simulink model "transfer_function_calculation"  (R2016a)
settings: Solver=VariableStepAuto  StartTime=0.0  StopTime=5  RelTol=1e-3
values from neighbouring files (symbols this model uses):
  a = .7    (= 0.7)    [PM_1_5MW_syn_27.m]
  Flux = 5.8264    [PM_1_5MW_syn_27.m]
  Id_set = 500    [PM_1_5MW_syn_27.m]
  Iq_set = -2200    [PM_1_5MW_syn_27.m]
  L = .0001    (= 0.0001)    [PM_1_5MW_syn_27.m]
  Ld = 0.001575    [PM_1_5MW_syn_27.m]
  Lq = 0.001575    [PM_1_5MW_syn_27.m]
  mn = 60000    [PM_1_5MW_syn_27.m]
  p = 26    [PM_1_5MW_syn_27.m]
  Rs = 0.000821    [PM_1_5MW_syn_27.m]
  Sollkurve_M_Optimum = [0 57121 101549 158670 228485 310994 406196 514092 634681 767965 810425 823386 ... (13 elements, 13x1)]    [Lookup_M_n.mat]
  Sollkurve_nGen_Optimum = [0 5 7 9 11 12 14 16 18 20 20.07 20.2 ... (13 elements, 13x1)]    [Lookup_M_n.mat]
  Speed_set = w_m    (= 2.10172548525)    [PM_1_5MW_syn_27.m]
  Ts_Power = 5.000000000000000e-06    (= 5e-06)    [PM_1_5MW_syn_27.m]
  Vdc = 1200    [PM_1_5MW_syn_27.m]
  Vh = Vm/6*0    (= 0)    [PM_1_5MW_syn_27.m]
undefined symbols (not defined in the file or in its folder): C2, Esw_Erec, Esw_Off, Esw_On, Page_Temp_C
undefined symbols (not defined in the file): Ts_Control, z
libraries: fl_lib x84, powerlib_meascontrol x58, simulink x56, nesl_utility x36, powerlib x33, simulink_extras x11
(part 3 of 6)

== system transfer_function_calculation/Generator/Generator /power calculation ==
  vdq : Inport
  idq : Inport  Port=2
  Complex to Magnitude-Angle : ComplexToMagnitudeAngle
  Complex to Real-Imag : ComplexToRealImag
  Demux : Demux  Outputs=2
  Demux1 : Demux  Outputs=2
  Gain : Gain  Gain=180/pi
  Gain1 : Gain  Gain=-1
  Gain4 : Gain  Gain=3/2
  Product2 : Product  RndMeth=Zero
  Real-Imag to Complex : RealImagToComplex
  Real-Imag to Complex1 : RealImagToComplex
  Trigonometric Function : Trigonometry  Operator=cos
  apparent power : Outport
  active power : Outport  Port=2
  reactive power : Outport  Port=3
  phi : Outport  Port=4
  cos phi : Outport  Port=5
  wires:
  Demux/1 -> Real-Imag to Complex/1
  Demux/2 -> Real-Imag to Complex/2
  Demux1/1 -> Real-Imag to Complex1/1
  Real-Imag to Complex/1 -> Product2/1
  Real-Imag to Complex1/1 -> Product2/2
  Product2/1 -> Gain4/1
  vdq/1 -> Demux/1
  idq/1 -> Demux1/1
  Complex to Magnitude-Angle/1 -> apparent power/1
  Complex to Magnitude-Angle/2 -> Trigonometric Function/1, Gain/1
  Gain/1 -> phi/1
  Demux1/2 -> Gain1/1
  Gain1/1 -> Real-Imag to Complex1/2
  Trigonometric Function/1 -> cos phi/1
  Complex to Real-Imag/1 -> active power/1
  Complex to Real-Imag/2 -> reactive power/1
  Gain4/1 -> Complex to Real-Imag/1, Complex to Magnitude-Angle/1

== system transfer_function_calculation/Generator/Generator Controller /Id controller ==
  Id_set : Inport
  Id_meas : Inport  Port=2
  Step : Step  Before=1  SampleTime=0
  Sum2 : Sum  Inputs=|-+
  Transfer Fcn (with initial states)1 : simulink_extras/Additional Linear/Transfer Fcn (with initial states)  N=[1 2888 714941]*7.50  D=[1 5626 5375320]  X0=0
  id : Scope  NumInputPorts=2
  id1 : Scope
  Vd_ref : Outport
  wires:
  Id_set/1 -> id/2, id1/1, Sum2/2
  Sum2/1 -> Transfer Fcn (with initial states)1/1
  Id_meas/1 -> id/1, Sum2/1
  Transfer Fcn (with initial states)1/1 -> Vd_ref/1

== system transfer_function_calculation/Generator/Generator Controller /Inverse Clarke Transformation ==
  ab : Inport
  Demux : Demux  Outputs=2
  Gain1 : Gain  Gain=1/2
  Gain2 : Gain  Gain=sqrt(3)
  Gain4 : Gain  Gain=1/2
  Mux : Mux  Inputs=3
  Sum : Sum  Inputs=|-+
  Sum1 : Sum  Inputs=|--
  abc : Outport
  wires:
  Mux/1 -> abc/1
  ab/1 -> Demux/1
  Sum1/1 -> Gain1/1
  Sum/1 -> Gain4/1
  Gain2/1 -> Sum1/2, Sum/2
  Demux/1 -> Sum1/1, Sum/1, Mux/1
  Demux/2 -> Gain2/1
  Gain4/1 -> Mux/2
  Gain1/1 -> Mux/3

== system transfer_function_calculation/Generator/Generator Controller /Inverse Park Transformation ==
  dq : Inport
  angle : Inport  Port=2
  Demux : Demux  Outputs=2
  Mux : Mux  Inputs=2
  Product{,1..3} (4 alike) : Product  RndMeth=Zero
  Sum : Sum  Inputs=|+-
  Sum1 : Sum  Inputs=|++
  cosine : Trigonometry  Operator=cos
  sine : Trigonometry
  ab : Outport
  wires:
  Sum1/1 -> Mux/2
  Sum/1 -> Mux/1
  Product2/1 -> Sum/2
  Product1/1 -> Sum/1
  Product3/1 -> Sum1/2
  Product/1 -> Sum1/1
  angle/1 -> cosine/1, sine/1
  cosine/1 -> Product3/2, Product1/2
  sine/1 -> Product2/2, Product/2
  Demux/2 -> Product3/1, Product2/1
  Demux/1 -> Product1/1, Product/1
  Mux/1 -> ab/1
  dq/1 -> Demux/1

== system transfer_function_calculation/Generator/Generator Controller /Iq controller ==
  Iq_meas : Inport
  Iq_set : Inport  Port=2
  Sum1 : Sum  Inputs=|-+
  Transfer Fcn (with initial states)1 : simulink_extras/Additional Linear/Transfer Fcn (with initial states)  N=[1 2888 714941]*7.50  D=[1 5626 5375320]  X0=0
  iq : Scope  NumInputPorts=2
  iq1 : Scope
  Vq_ref : Outport
  wires:
  Iq_set/1 -> iq/1, Sum1/2
  Sum1/1 -> Transfer Fcn (with initial states)1/1
  Iq_meas/1 -> iq1/1, iq/2, Sum1/1
  Transfer Fcn (with initial states)1/1 -> Vq_ref/1

== system transfer_function_calculation/Generator/Generator Controller /Parktransformation ==
  i_abc : Inport
  theta : Inport  Port=2
  3phase to ab : Subsystem
  Cartesian to Polar : simulink_extras/Transformations/Cartesian to Polar
  Demux : Demux  Outputs=2
  Display : Display
  Display1 : Display
  Scope : Scope  NumInputPorts=3
  Scope1 : Scope  NumInputPorts=3
  Scope2 : Scope  NumInputPorts=3
  alpha-beta to dq : Subsystem
  i_dq : Outport
  wires:
  3phase to ab/1(Out1) -> Scope/2, Demux/1, alpha-beta to dq/2("alpha-beta ")
  alpha-beta to dq/1(Out1) -> Scope/1, i_dq/1
  i_abc/1 -> Scope1/1, 3phase to ab/1(In1)
  theta/1 -> Scope/3, alpha-beta to dq/1(theta)
  Demux/1 -> Cartesian to Polar/1
  Demux/2 -> Cartesian to Polar/2
  Cartesian to Polar/1 -> Scope2/1, Display/1
  Cartesian to Polar/2 -> Scope2/2, Display1/1

== system transfer_function_calculation/Generator/Generator Controller /Speed Controller ==
  meas : Inport
  set : Inport  Port=2
  PID Controller1 : simulink/Continuous/PID Controller  Controller=PI  TimeDomain=Continuous-time  SampleTime=-1  IntegratorMethod=Forward Euler  FilterMethod=Forward Euler  Form=Parallel  UseFilter=on  ControllerParametersSource=internal  P=5437  I=1000000  D=0  N=100  InitialConditionSource=internal  InitialConditionForIntegrator=0  InitialConditionForFilter=0  ExternalReset=none  LimitOutput=off  UpperSaturationLimit=inf  LowerSaturationLimit=-inf  LinearizeAsGain=on  AntiWindupMode=none  Kb=1  TrackingMode=off  Kt=1  PParamMin=[]  PParamMax=[]  IParamMin=[]  IParamMax=[]  DParamMin=[]  DParamMax=[]  NParamMin=[]  NParamMax=[]  KbParamMin=[]  KbParamMax=[]  KtParamMin=[]  KtParamMax=[]  POutMin=[]  POutMax=[]  IOutMin=[]  IOutMax=[]  DOutMin=[]  DOutMax=[]  NOutMin=[]  NOutMax=[]  KbOutMin=[]  KbOutMax=[]  KtOutMin=[]  KtOutMax=[]  IntegratorOutMin=[]  IntegratorOutMax=[]  FilterOutMin=[]  FilterOutMax=[]  SumOutMin=[]  SumOutMax=[]  SumI1OutMin=[]  SumI1OutMax=[]  SumI2OutMin=[]  SumI2OutMax=[]  SumI3OutMin=[]  SumI3OutMax=[]  SumDOutMin=[]  SumDOutMax=[]  SaturationOutMin=[]  SaturationOutMax=[]  IntegratorContinuousStateAttributes=''  IntegratorStateMustResolveToSignalObject=off  IntegratorRTWStateStorageClass=Auto  FilterContinuousStateAttributes=''  FilterStateMustResolveToSignalObject=off  FilterRTWStateStorageClass=Auto  DifferentiatorICPrevScaledInput=0  DifferentiatorOutMin=[]  DifferentiatorOutMax=[]
  Sum1 : Sum  Inputs=|-+
  Transfer Fcn (with initial states)1 : simulink_extras/Additional Linear/Transfer Fcn (with initial states)  Commented=on  N=[18.688 3793]  D=[1 3808]  X0=0
  "speed " : Scope  NumInputPorts=2
  speed 1 : Scope
  Act : Outport
  wires:
  set/1 -> "speed "/1, Sum1/2
  meas/1 -> "speed "/2, speed 1/1, Sum1/1
  Sum1/1 -> PID Controller1/1
  PID Controller1/1 -> Act/1

== system transfer_function_calculation/Generator/Modulation index2/Clarke transformation ==
  In1 : Inport
  Demux : Demux  Outputs=3
  Gain3 : Gain  Gain=1/sqrt(3)
  Mux : Mux  Inputs=2
  Scope : Scope
  Sum1 : Sum  Inputs=|+-
  Out1 : Outport
  wires:
  Gain3/1 -> Mux/2
  Demux/1 -> Mux/1
  In1/1 -> Demux/1
  Sum1/1 -> Gain3/1
  Demux/3 -> Sum1/2
  Demux/2 -> Sum1/1
  Mux/1 -> Out1/1, Scope/1

== system transfer_function_calculation/Generator/3 Level Converter2/Loss Calculation/Leg A1 ==
  G : Inport  PortDimensions=2
  G1 : Inport  Port=2  PortDimensions=2
  Ambient Temperature (C) : Constant  Value=40
  Heat Sink (Simscape thermal model) : Subsystem  mask(Simscape Thermal model (2-cell Cauer network)){Rth=[ 0.02  0.072 ], Cth=[ 5  10 ]/10, Tinit=123}
      mask prompts: Rth "Thermal resistances  [case-to-sink  sink-to-ambient ] (K/W):"; Cth "Thermal capacitances  [case  sink ] (J/K):"; Tinit "Initial temperature (degrees Celsisus)"
  Scope : Scope
  Scope1 : Scope
  Subsystem : Subsystem
  Tsink : Scope
  m : Outport
  wires:
  G/1 -> Subsystem/1(In1), Scope/1
  G1/1 -> Scope1/1, Subsystem/2(In2)
  Ambient Temperature (C)/1 -> Heat Sink (Simscape thermal model)/1(Ta)
  Heat Sink (Simscape thermal model)/1(Tsink) -> Tsink/1
  Subsystem/1(Out1) -> m/1
  connections:
  Heat Sink (Simscape thermal model)/RConn1 -- Subsystem/LConn1

== system transfer_function_calculation/Generator/3 Level Converter2/Loss Calculation/Leg A2 ==
  G : Inport  PortDimensions=2
  G1 : Inport  Port=2  PortDimensions=2
  Ambient Temperature (C) : Constant  Value=40
  Heat Sink (Simscape thermal model) : Subsystem  mask(Simscape Thermal model (2-cell Cauer network)){Rth=[ 0.02  0.072 ], Cth=[ 1  5 ]/10, Tinit=123}
      mask prompts: Rth "Thermal resistances  [case-to-sink  sink-to-ambient ] (K/W):"; Cth "Thermal capacitances  [case  sink ] (J/K):"; Tinit "Initial temperature (degrees Celsisus)"
  Scope : Scope
  Scope1 : Scope
  Subsystem : Subsystem
  Tsink : Scope
  m : Outport
  wires:
  Subsystem/1(Out1) -> m/1
  Heat Sink (Simscape thermal model)/1(Tsink) -> Tsink/1
  Ambient Temperature (C)/1 -> Heat Sink (Simscape thermal model)/1(Ta)
  G1/1 -> Subsystem/2(In2), Scope1/1
  G/1 -> Scope/1, Subsystem/1(In1)
  connections:
  Heat Sink (Simscape thermal model)/RConn1 -- Subsystem/LConn1

== system transfer_function_calculation/Generator/3 Level Converter2/Loss Calculation/Leg B1 ==
  G : Inport  PortDimensions=2
  G1 : Inport  Port=2  PortDimensions=2
  Ambient Temperature (C) : Constant  Value=40
  Heat Sink (Simscape thermal model) : Subsystem  mask(Simscape Thermal model (2-cell Cauer network)){Rth=[ 0.02  0.072 ], Cth=[ 1  5 ]/10, Tinit=123}
      mask prompts: Rth "Thermal resistances  [case-to-sink  sink-to-ambient ] (K/W):"; Cth "Thermal capacitances  [case  sink ] (J/K):"; Tinit "Initial temperature (degrees Celsisus)"
  Scope : Scope
  Scope1 : Scope
  Subsystem : Subsystem
  Tsink : Scope
  m : Outport
  wires:
  G/1 -> Subsystem/1(In1), Scope/1
  G1/1 -> Scope1/1, Subsystem/2(In2)
  Ambient Temperature (C)/1 -> Heat Sink (Simscape thermal model)/1(Ta)
  Heat Sink (Simscape thermal model)/1(Tsink) -> Tsink/1
  Subsystem/1(Out1) -> m/1
  connections:
  Heat Sink (Simscape thermal model)/RConn1 -- Subsystem/LConn1

== system transfer_function_calculation/Generator/3 Level Converter2/Loss Calculation/Leg B2 ==
  G : Inport  PortDimensions=2
  G1 : Inport  Port=2  PortDimensions=2
  Ambient Temperature (C) : Constant  Value=40
  Heat Sink (Simscape thermal model) : Subsystem  mask(Simscape Thermal model (2-cell Cauer network)){Rth=[ 0.02  0.072 ], Cth=[ 1  5 ]/10, Tinit=123}
      mask prompts: Rth "Thermal resistances  [case-to-sink  sink-to-ambient ] (K/W):"; Cth "Thermal capacitances  [case  sink ] (J/K):"; Tinit "Initial temperature (degrees Celsisus)"
  Scope : Scope
  Scope1 : Scope
  Subsystem : Subsystem
  Tsink : Scope
  m : Outport
  wires:
  Subsystem/1(Out1) -> m/1
  Heat Sink (Simscape thermal model)/1(Tsink) -> Tsink/1
  Ambient Temperature (C)/1 -> Heat Sink (Simscape thermal model)/1(Ta)
  G1/1 -> Subsystem/2(In2), Scope1/1
  G/1 -> Scope/1, Subsystem/1(In1)
  connections:
  Heat Sink (Simscape thermal model)/RConn1 -- Subsystem/LConn1

== system transfer_function_calculation/Generator/3 Level Converter2/Loss Calculation/Leg C1 ==
  G : Inport  PortDimensions=2
  G1 : Inport  Port=2  PortDimensions=2
  Ambient Temperature (C) : Constant  Value=40
  Heat Sink (Simscape thermal model) : Subsystem  mask(Simscape Thermal model (2-cell Cauer network)){Rth=[ 0.02  0.072 ], Cth=[ 1  5 ]/10, Tinit=123}
      mask prompts: Rth "Thermal resistances  [case-to-sink  sink-to-ambient ] (K/W):"; Cth "Thermal capacitances  [case  sink ] (J/K):"; Tinit "Initial temperature (degrees Celsisus)"
  Scope : Scope
  Scope1 : Scope
  Subsystem : Subsystem
  Tsink : Scope
  m : Outport
  wires:
  G/1 -> Subsystem/1(In1), Scope/1
  G1/1 -> Scope1/1, Subsystem/2(In2)
  Ambient Temperature (C)/1 -> Heat Sink (Simscape thermal model)/1(Ta)
  Heat Sink (Simscape thermal model)/1(Tsink) -> Tsink/1
  Subsystem/1(Out1) -> m/1
  connections:
  Heat Sink (Simscape thermal model)/RConn1 -- Subsystem/LConn1

== system transfer_function_calculation/Generator/3 Level Converter2/Loss Calculation/Leg C2 ==
  G : Inport  PortDimensions=2
  G1 : Inport  Port=2  PortDimensions=2
  Ambient Temperature (C) : Constant  Value=40
  Heat Sink (Simscape thermal model) : Subsystem  mask(Simscape Thermal model (2-cell Cauer network)){Rth=[ 0.02  0.072 ], Cth=[ 1  5 ]/10, Tinit=123}
      mask prompts: Rth "Thermal resistances  [case-to-sink  sink-to-ambient ] (K/W):"; Cth "Thermal capacitances  [case  sink ] (J/K):"; Tinit "Initial temperature (degrees Celsisus)"
  Scope : Scope
  Scope1 : Scope
  Subsystem : Subsystem
  Tsink : Scope
  m : Outport
  wires:
  Subsystem/1(Out1) -> m/1
  Heat Sink (Simscape thermal model)/1(Tsink) -> Tsink/1
  Ambient Temperature (C)/1 -> Heat Sink (Simscape thermal model)/1(Ta)
  G1/1 -> Subsystem/2(In2), Scope1/1
  G/1 -> Scope/1, Subsystem/1(In1)
  connections:
  Heat Sink (Simscape thermal model)/RConn1 -- Subsystem/LConn1

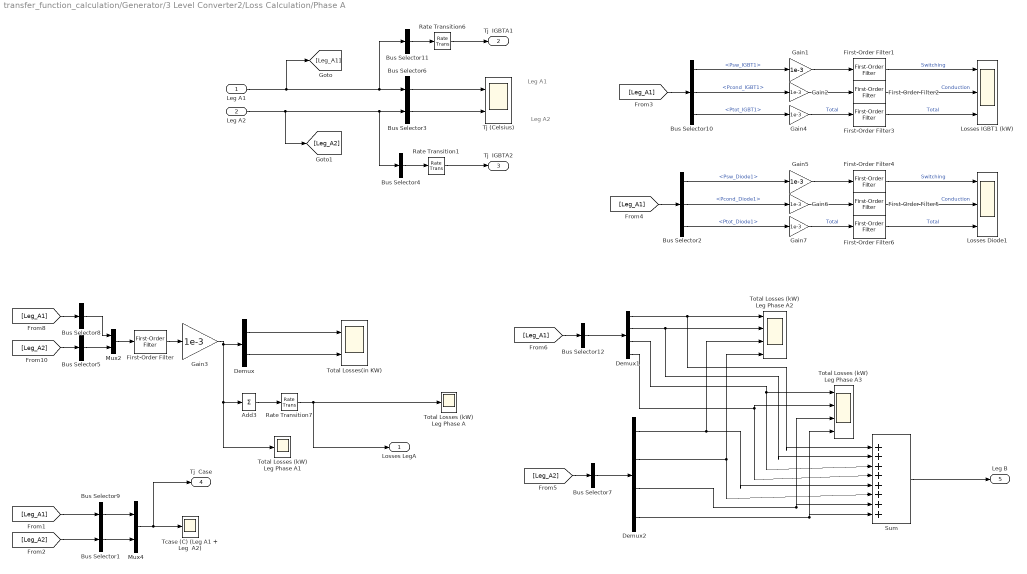
== system transfer_function_calculation/Generator/3 Level Converter2/Loss Calculation/Phase A ==
  note: Leg A2
  note: Leg A1
  Leg A1 : Inport
  Leg A2 : Inport  Port=2
  Add3 : Sum  Inputs=+
  Bus Selector1 : BusSelector  OutputSignals=Tcase  OutputAsBus=on
  Bus Selector10 : BusSelector  OutputSignals=Psw_IGBT1,Pcond_IGBT1,Ptot_IGBT1
  Bus Selector11 : BusSelector  OutputSignals=Tj_IGBT1  OutputAsBus=on
  Bus Selector{5,7..8,12} (4 alike) : BusSelector  OutputSignals=Ptot_IGBT1,Ptot_IGBT2,Ptot_Diode1,Ptot_Diode2  OutputAsBus=on
  Bus Selector2 : BusSelector  OutputSignals=Psw_Diode1,Pcond_Diode1,Ptot_Diode1
  Bus Selector3 : BusSelector  OutputSignals=Tj_IGBT1,Tj_IGBT2,Tj_Diode1,Tj_Diode2  OutputAsBus=on
  Bus Selector4 : BusSelector  OutputSignals=Tj_IGBT1  OutputAsBus=on
  Bus Selector6 : BusSelector  OutputSignals=Tj_IGBT1,Tj_IGBT2,Tj_Diode1,Tj_Diode2  OutputAsBus=on
  Bus Selector9 : BusSelector  OutputSignals=Tcase  OutputAsBus=on
  Demux : Demux  Outputs=2
  Demux1 : Demux
  Demux2 : Demux
  First-Order Filter{,1..6} (7 alike) : powerlib_meascontrol/Filters/First-Order Filter  FilterType=Lowpass  Tc=100e-3  Ts=Ts_Power  Initialize=off  Vac_Init=[0, 0, 60]  Vdc_Init=0  PlotResponse=off  FreqRange="[0,  200,  1]"
  Gain{1..7} (7 alike) : Gain  Gain=1e-3
  Losses Diode1 : Scope  NumInputPorts=3
  "Losses IGBT1 (kW) " : Scope  NumInputPorts=3
  Mux2 : Mux  Inputs=2
  Mux4 : Mux  Inputs=2
  Rate Transition1 : RateTransition  OutPortSampleTime=Ts_Control
  Rate Transition6 : RateTransition  OutPortSampleTime=Ts_Control
  Rate Transition7 : RateTransition  OutPortSampleTime=Ts_Control
  Sum : Sum  Inputs=|++++++++
  Tcase (C) (Leg A1 + Leg  A2) : Scope
  Tj (Celsius) : Scope  NumInputPorts=2
  Total Losses (kW) Leg Phase A : Scope
  Total Losses (kW) Leg Phase A1 : Scope
  Total Losses (kW) Leg Phase A2 : Scope  NumInputPorts=4
  Total Losses (kW) Leg Phase A3 : Scope  NumInputPorts=4
  Total Losses(in KW) : Scope  NumInputPorts=2
  Losses LegA : Outport
  Tj  IGBTA1 : Outport  Port=2
  Tj  IGBTA2 : Outport  Port=3
  Tj  Case : Outport  Port=4
  Leg B : Outport  Port=5
  wires:
  Bus Selector10/1 -> Gain1/1  "<Psw_IGBT1>"
  [Leg_A2] -> Bus Selector5/1
  Bus Selector8/1 -> Mux2/1
  Bus Selector9/1 -> Mux4/1
  Bus Selector5/1 -> Mux2/2
  Gain3/1 -> Total Losses (kW) Leg Phase A1/1, Add3/1, Demux/1
  [Leg_A1] -> Bus Selector8/1
  Add3/1 -> Rate Transition7/1
  [Leg_A2] -> Bus Selector1/1
  Bus Selector1/1 -> Mux4/2
  Bus Selector10/2 -> Gain2/1  "<Pcond_IGBT1>"
  Mux4/1 -> Tj  Case/1, Tcase (C) (Leg A1 + Leg  A2)/1
  Bus Selector10/3 -> Gain4/1  "<Ptot_IGBT1>"
  First-Order Filter1/1 -> "Losses IGBT1 (kW) "/1  "Switching"
  Bus Selector6/1 -> Tj (Celsius)/1
  [Leg_A1] -> Bus Selector10/1
  First-Order Filter2/1 -> "Losses IGBT1 (kW) "/2  "Conduction"
  Mux2/1 -> First-Order Filter/1
  First-Order Filter/1 -> Gain3/1
  [Leg_A1] -> Bus Selector9/1
  Bus Selector3/1 -> Tj (Celsius)/2
  Gain2/1 -> First-Order Filter2/1
  Gain1/1 -> First-Order Filter1/1
  Bus Selector11/1 -> Rate Transition6/1
  Rate Transition6/1 -> Tj  IGBTA1/1
  Gain4/1 -> First-Order Filter3/1  "Total"
  Rate Transition7/1 -> Losses LegA/1, Total Losses (kW) Leg Phase A/1
  First-Order Filter3/1 -> "Losses IGBT1 (kW) "/3  "Total"
  Leg A1/1 -> [Leg_A1], Bus Selector11/1, Bus Selector6/1
  Bus Selector4/1 -> Rate Transition1/1
  Rate Transition1/1 -> Tj  IGBTA2/1
  Leg A2/1 -> [Leg_A2], Bus Selector4/1, Bus Selector3/1
  Demux/2 -> Total Losses(in KW)/2
  Demux/1 -> Total Losses(in KW)/1
  Bus Selector2/1 -> Gain5/1  "<Psw_Diode1>"
  Bus Selector2/2 -> Gain6/1  "<Pcond_Diode1>"
  Bus Selector2/3 -> Gain7/1  "<Ptot_Diode1>"
  First-Order Filter4/1 -> Losses Diode1/1  "Switching"
  [Leg_A1] -> Bus Selector2/1
  First-Order Filter5/1 -> Losses Diode1/2  "Conduction"
  Gain6/1 -> First-Order Filter5/1
  Gain5/1 -> First-Order Filter4/1
  Gain7/1 -> First-Order Filter6/1  "Total"
  First-Order Filter6/1 -> Losses Diode1/3  "Total"
  [Leg_A2] -> Bus Selector7/1
  [Leg_A1] -> Bus Selector12/1
  Bus Selector12/1 -> Demux1/1
  Demux1/1 -> Sum/1, Total Losses (kW) Leg Phase A2/1
  Demux1/2 -> Sum/2, Total Losses (kW) Leg Phase A2/2
  Demux1/3 -> Total Losses (kW) Leg Phase A3/1, Sum/3
  Bus Selector7/1 -> Demux2/1
  Demux2/1 -> Total Losses (kW) Leg Phase A2/3, Sum/5
  Demux2/2 -> Total Losses (kW) Leg Phase A2/4, Sum/6
  Demux2/3 -> Total Losses (kW) Leg Phase A3/3, Sum/7
  Demux2/4 -> Sum/8, Total Losses (kW) Leg Phase A3/4
  Sum/1 -> Leg B/1
  Demux1/4 -> Sum/4, Total Losses (kW) Leg Phase A3/2

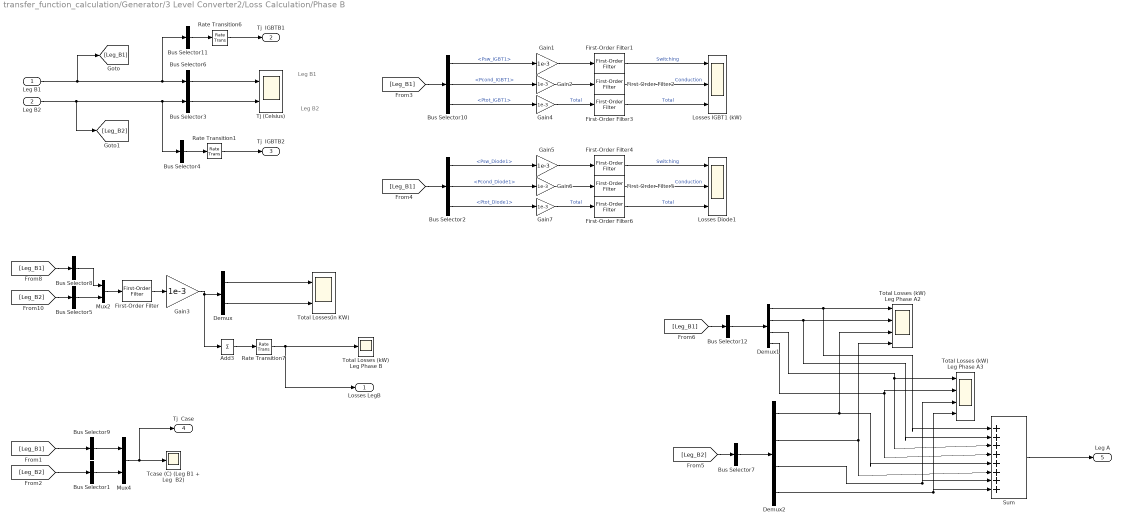
== system transfer_function_calculation/Generator/3 Level Converter2/Loss Calculation/Phase B ==
  note: Leg B1
  note: Leg B2
  Leg B1 : Inport
  Leg B2 : Inport  Port=2
  Add3 : Sum  Inputs=+
  Bus Selector1 : BusSelector  OutputSignals=Tcase  OutputAsBus=on
  Bus Selector10 : BusSelector  OutputSignals=Psw_IGBT1,Pcond_IGBT1,Ptot_IGBT1
  Bus Selector11 : BusSelector  OutputSignals=Tj_IGBT1  OutputAsBus=on
  Bus Selector{5,7..8,12} (4 alike) : BusSelector  OutputSignals=Ptot_IGBT1,Ptot_IGBT2,Ptot_Diode1,Ptot_Diode2  OutputAsBus=on
  Bus Selector2 : BusSelector  OutputSignals=Psw_Diode1,Pcond_Diode1,Ptot_Diode1
  Bus Selector3 : BusSelector  OutputSignals=Tj_IGBT1,Tj_IGBT2,Tj_Diode1,Tj_Diode2  OutputAsBus=on
  Bus Selector4 : BusSelector  OutputSignals=Tj_IGBT1  OutputAsBus=on
  Bus Selector6 : BusSelector  OutputSignals=Tj_IGBT1,Tj_IGBT2,Tj_Diode1,Tj_Diode2  OutputAsBus=on
  Bus Selector9 : BusSelector  OutputSignals=Tcase  OutputAsBus=on
  Demux : Demux  Outputs=2
  Demux1 : Demux
  Demux2 : Demux
  First-Order Filter{,1..6} (7 alike) : powerlib_meascontrol/Filters/First-Order Filter  FilterType=Lowpass  Tc=100e-3  Ts=Ts_Power  Initialize=off  Vac_Init=[0, 0, 60]  Vdc_Init=0  PlotResponse=off  FreqRange="[0,  200,  1]"
  Gain{1..7} (7 alike) : Gain  Gain=1e-3
  Losses Diode1 : Scope  NumInputPorts=3
  "Losses IGBT1 (kW) " : Scope  NumInputPorts=3
  Mux2 : Mux  Inputs=2
  Mux4 : Mux  Inputs=2
  Rate Transition1 : RateTransition  OutPortSampleTime=Ts_Control
  Rate Transition6 : RateTransition  OutPortSampleTime=Ts_Control
  Rate Transition7 : RateTransition  OutPortSampleTime=Ts_Control
  Sum : Sum  Inputs=|++++++++
  Tcase (C) (Leg B1 + Leg  B2) : Scope
  Tj (Celsius) : Scope  NumInputPorts=2
  Total Losses (kW) Leg Phase A2 : Scope  NumInputPorts=4
  Total Losses (kW) Leg Phase A3 : Scope  NumInputPorts=4
  Total Losses (kW) Leg Phase B : Scope
  Total Losses(in KW) : Scope  NumInputPorts=2
  Losses LegB : Outport
  Tj  IGBTB1 : Outport  Port=2
  Tj  IGBTB2 : Outport  Port=3
  Tj  Case : Outport  Port=4
  Leg A : Outport  Port=5
  wires:
  First-Order Filter6/1 -> Losses Diode1/3  "Total"
  Gain7/1 -> First-Order Filter6/1  "Total"
  Gain5/1 -> First-Order Filter4/1
  Gain6/1 -> First-Order Filter5/1
  First-Order Filter5/1 -> Losses Diode1/2  "Conduction"
  [Leg_B1] -> Bus Selector2/1
  First-Order Filter4/1 -> Losses Diode1/1  "Switching"
  Bus Selector2/3 -> Gain7/1  "<Ptot_Diode1>"
  Bus Selector2/2 -> Gain6/1  "<Pcond_Diode1>"
  Bus Selector2/1 -> Gain5/1  "<Psw_Diode1>"
  Demux/1 -> Total Losses(in KW)/1
  Demux/2 -> Total Losses(in KW)/2
  Leg B2/1 -> Bus Selector3/1, Bus Selector4/1, [Leg_B2]
  Rate Transition1/1 -> Tj  IGBTB2/1
  Bus Selector4/1 -> Rate Transition1/1
  Leg B1/1 -> Bus Selector6/1, Bus Selector11/1, [Leg_B1]
  First-Order Filter3/1 -> "Losses IGBT1 (kW) "/3  "Total"
  Rate Transition7/1 -> Total Losses (kW) Leg Phase B/1, Losses LegB/1
  Gain4/1 -> First-Order Filter3/1  "Total"
  Rate Transition6/1 -> Tj  IGBTB1/1
  Bus Selector11/1 -> Rate Transition6/1
  Gain1/1 -> First-Order Filter1/1
  Gain2/1 -> First-Order Filter2/1
  Bus Selector3/1 -> Tj (Celsius)/2
  [Leg_B1] -> Bus Selector9/1
  First-Order Filter/1 -> Gain3/1
  Mux2/1 -> First-Order Filter/1
  First-Order Filter2/1 -> "Losses IGBT1 (kW) "/2  "Conduction"
  [Leg_B1] -> Bus Selector10/1
  Bus Selector6/1 -> Tj (Celsius)/1
  First-Order Filter1/1 -> "Losses IGBT1 (kW) "/1  "Switching"
  Bus Selector10/3 -> Gain4/1  "<Ptot_IGBT1>"
  Mux4/1 -> Tcase (C) (Leg B1 + Leg  B2)/1, Tj  Case/1
  Bus Selector10/2 -> Gain2/1  "<Pcond_IGBT1>"
  Bus Selector1/1 -> Mux4/2
  [Leg_B2] -> Bus Selector1/1
  Add3/1 -> Rate Transition7/1
  [Leg_B1] -> Bus Selector8/1
  Gain3/1 -> Demux/1, Add3/1
  Bus Selector5/1 -> Mux2/2
  Bus Selector9/1 -> Mux4/1
  Bus Selector8/1 -> Mux2/1
  [Leg_B2] -> Bus Selector5/1
  Bus Selector10/1 -> Gain1/1  "<Psw_IGBT1>"
  [Leg_B2] -> Bus Selector7/1
  [Leg_B1] -> Bus Selector12/1
  Bus Selector12/1 -> Demux1/1
  Demux1/1 -> Sum/1, Total Losses (kW) Leg Phase A2/1
  Demux1/2 -> Sum/2, Total Losses (kW) Leg Phase A2/2
  Demux1/3 -> Total Losses (kW) Leg Phase A3/1, Sum/3
  Bus Selector7/1 -> Demux2/1
  Demux2/1 -> Total Losses (kW) Leg Phase A2/3, Sum/5
  Demux2/2 -> Total Losses (kW) Leg Phase A2/4, Sum/6
  Demux2/3 -> Total Losses (kW) Leg Phase A3/3, Sum/7
  Demux2/4 -> Sum/8, Total Losses (kW) Leg Phase A3/4
  Demux1/4 -> Sum/4, Total Losses (kW) Leg Phase A3/2
  Sum/1 -> Leg A/1

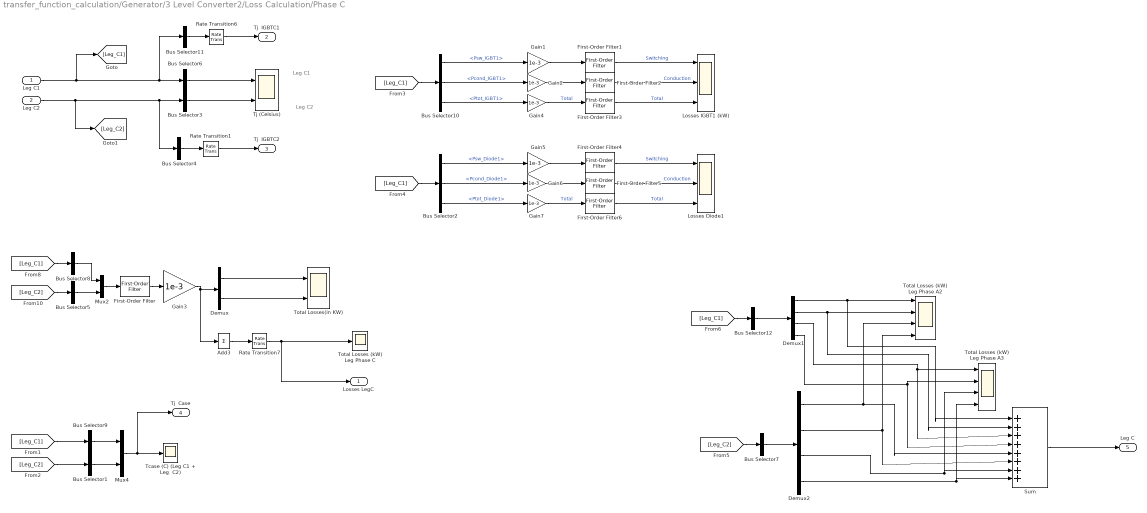
== system transfer_function_calculation/Generator/3 Level Converter2/Loss Calculation/Phase C ==
  note: Leg C2
  note: Leg C1
  Leg C1 : Inport
  Leg C2 : Inport  Port=2
  Add3 : Sum  Inputs=+
  Bus Selector1 : BusSelector  OutputSignals=Tcase  OutputAsBus=on
  Bus Selector10 : BusSelector  OutputSignals=Psw_IGBT1,Pcond_IGBT1,Ptot_IGBT1
  Bus Selector11 : BusSelector  OutputSignals=Tj_IGBT1  OutputAsBus=on
  Bus Selector{5,7..8,12} (4 alike) : BusSelector  OutputSignals=Ptot_IGBT1,Ptot_IGBT2,Ptot_Diode1,Ptot_Diode2  OutputAsBus=on
  Bus Selector2 : BusSelector  OutputSignals=Psw_Diode1,Pcond_Diode1,Ptot_Diode1
  Bus Selector3 : BusSelector  OutputSignals=Tj_IGBT1,Tj_IGBT2,Tj_Diode1,Tj_Diode2  OutputAsBus=on
  Bus Selector4 : BusSelector  OutputSignals=Tj_IGBT1  OutputAsBus=on
  Bus Selector6 : BusSelector  OutputSignals=Tj_IGBT1,Tj_IGBT2,Tj_Diode1,Tj_Diode2  OutputAsBus=on
  Bus Selector9 : BusSelector  OutputSignals=Tcase  OutputAsBus=on
  Demux : Demux  Outputs=2
  Demux1 : Demux
  Demux2 : Demux
  First-Order Filter{,1..6} (7 alike) : powerlib_meascontrol/Filters/First-Order Filter  FilterType=Lowpass  Tc=100e-3  Ts=Ts_Power  Initialize=off  Vac_Init=[0, 0, 60]  Vdc_Init=0  PlotResponse=off  FreqRange="[0,  200,  1]"
  Gain{1..7} (7 alike) : Gain  Gain=1e-3
  Losses Diode1 : Scope  NumInputPorts=3
  "Losses IGBT1 (kW) " : Scope  NumInputPorts=3
  Mux2 : Mux  Inputs=2
  Mux4 : Mux  Inputs=2
  Rate Transition1 : RateTransition  OutPortSampleTime=Ts_Control
  Rate Transition6 : RateTransition  OutPortSampleTime=Ts_Control
  Rate Transition7 : RateTransition  OutPortSampleTime=Ts_Control
  Sum : Sum  Inputs=|++++++++
  Tcase (C) (Leg C1 + Leg  C2) : Scope
  Tj (Celsius) : Scope  NumInputPorts=2
  Total Losses (kW) Leg Phase A2 : Scope  NumInputPorts=4
  Total Losses (kW) Leg Phase A3 : Scope  NumInputPorts=4
  Total Losses (kW) Leg Phase C : Scope
  Total Losses(in KW) : Scope  NumInputPorts=2
  Losses LegC : Outport
  Tj  IGBTC1 : Outport  Port=2
  Tj  IGBTC2 : Outport  Port=3
  Tj  Case : Outport  Port=4
  Leg C : Outport  Port=5
  wires:
  Bus Selector10/1 -> Gain1/1  "<Psw_IGBT1>"
  [Leg_C2] -> Bus Selector5/1
  Bus Selector8/1 -> Mux2/1
  Bus Selector9/1 -> Mux4/1
  Bus Selector5/1 -> Mux2/2
  Gain3/1 -> Add3/1, Demux/1
  [Leg_C1] -> Bus Selector8/1
  Add3/1 -> Rate Transition7/1
  [Leg_C2] -> Bus Selector1/1
  Bus Selector1/1 -> Mux4/2
  Bus Selector10/2 -> Gain2/1  "<Pcond_IGBT1>"
  Mux4/1 -> Tj  Case/1, Tcase (C) (Leg C1 + Leg  C2)/1
  Bus Selector10/3 -> Gain4/1  "<Ptot_IGBT1>"
  First-Order Filter1/1 -> "Losses IGBT1 (kW) "/1  "Switching"
  Bus Selector6/1 -> Tj (Celsius)/1
  [Leg_C1] -> Bus Selector10/1
  First-Order Filter2/1 -> "Losses IGBT1 (kW) "/2  "Conduction"
  Mux2/1 -> First-Order Filter/1
  First-Order Filter/1 -> Gain3/1
  [Leg_C1] -> Bus Selector9/1
  Bus Selector3/1 -> Tj (Celsius)/2
  Gain2/1 -> First-Order Filter2/1
  Gain1/1 -> First-Order Filter1/1
  Bus Selector11/1 -> Rate Transition6/1
  Rate Transition6/1 -> Tj  IGBTC1/1
  Gain4/1 -> First-Order Filter3/1  "Total"
  Rate Transition7/1 -> Losses LegC/1, Total Losses (kW) Leg Phase C/1
  First-Order Filter3/1 -> "Losses IGBT1 (kW) "/3  "Total"
  Leg C1/1 -> [Leg_C1], Bus Selector11/1, Bus Selector6/1
  Bus Selector4/1 -> Rate Transition1/1
  Rate Transition1/1 -> Tj  IGBTC2/1
  Leg C2/1 -> [Leg_C2], Bus Selector4/1, Bus Selector3/1
  Demux/2 -> Total Losses(in KW)/2
  Demux/1 -> Total Losses(in KW)/1
  Bus Selector2/1 -> Gain5/1  "<Psw_Diode1>"
  Bus Selector2/2 -> Gain6/1  "<Pcond_Diode1>"
  Bus Selector2/3 -> Gain7/1  "<Ptot_Diode1>"
  First-Order Filter4/1 -> Losses Diode1/1  "Switching"
  [Leg_C1] -> Bus Selector2/1
  First-Order Filter5/1 -> Losses Diode1/2  "Conduction"
  Gain6/1 -> First-Order Filter5/1
  Gain5/1 -> First-Order Filter4/1
  Gain7/1 -> First-Order Filter6/1  "Total"
  First-Order Filter6/1 -> Losses Diode1/3  "Total"
  [Leg_C2] -> Bus Selector7/1
  [Leg_C1] -> Bus Selector12/1
  Bus Selector12/1 -> Demux1/1
  Demux1/1 -> Sum/1, Total Losses (kW) Leg Phase A2/1
  Demux1/2 -> Sum/2, Total Losses (kW) Leg Phase A2/2
  Demux1/3 -> Total Losses (kW) Leg Phase A3/1, Sum/3
  Bus Selector7/1 -> Demux2/1
  Demux2/1 -> Total Losses (kW) Leg Phase A2/3, Sum/5
  Demux2/2 -> Total Losses (kW) Leg Phase A2/4, Sum/6
  Demux2/3 -> Total Losses (kW) Leg Phase A3/3, Sum/7
  Demux2/4 -> Sum/8, Total Losses (kW) Leg Phase A3/4
  Sum/1 -> Leg C/1
  Demux1/4 -> Sum/4, Total Losses (kW) Leg Phase A3/2

== system transfer_function_calculation/Generator/3 Level Converter2/SPWM Generator/ Comparator Phase B ==
  Ref signal : Inport
  3rd harmonic injection : Sin  Amplitude=Vh  Frequency=314*3  SampleTime=0
  Carrier wave +ve : simulink/Sources/Repeating Sequence  rep_seq_t=.0001*[0 2 4]  rep_seq_y=a*[2 0 2]
  Carrier wave -ve : simulink/Sources/Repeating Sequence  rep_seq_t=.0001*[0 2 4]  rep_seq_y=a*[0 -2 0]
  Mux : Mux  Inputs=3
  Relational Operator : RelationalOperator  Operator=>  OutDataTypeStr=fixdt(1,16)
  Relational Operator1 : RelationalOperator  Operator=>  OutDataTypeStr=boolean
  Scope : Scope
  Scope4 : Scope
  Scope5 : Scope  NumInputPorts=2
  Scope6 : Scope  NumInputPorts=3
  Sum : Sum  Inputs=|++
  Sum1 : Sum  Inputs=|+-
  Out1 : Outport
  wires:
  Relational Operator1/1 -> Scope6/3, Sum1/2
  Relational Operator/1 -> Sum1/1
  Carrier wave +ve/1 -> Mux/1, Relational Operator/2, Scope5/2
  Mux/1 -> Scope/1
  3rd harmonic injection/1 -> Sum/2
  Ref signal/1 -> Sum/1
  Carrier wave -ve/1 -> Mux/2, Relational Operator1/1, Scope6/1
  Sum/1 -> Mux/3, Relational Operator/1, Scope5/1, Relational Operator1/2, Scope6/2, Scope4/1
  Sum1/1 -> Out1/1

== system transfer_function_calculation/Generator/3 Level Converter2/SPWM Generator/Comparator Phase A ==
  "Ref Signal " : Inport
  3rd harmonic injection : Sin  Amplitude=Vh  Frequency=314*3  SampleTime=0
  Carrier wave +ve : simulink/Sources/Repeating Sequence  rep_seq_t=.0001*[0 2 4]  rep_seq_y=a*[2 0 2]
  Carrier wave -ve : simulink/Sources/Repeating Sequence  rep_seq_t=.0001*[0 2 4]  rep_seq_y="a*[0  -2  0]"
  Mux : Mux  Inputs=3
  Mux1 : Mux  Inputs=3
  Relational Operator : RelationalOperator  Operator=>  OutDataTypeStr=fixdt(1,16)
  Relational Operator1 : RelationalOperator  Operator=>  OutDataTypeStr=boolean
  Scope : Scope
  Scope1 : Scope
  Scope2 : Scope  NumInputPorts=2
  Scope3 : Scope  NumInputPorts=3
  Scope4 : Scope
  Scope5 : Scope  NumInputPorts=2
  Sum : Sum  Inputs=|++
  Sum1 : Sum  Inputs=|+-
  Out1 : Outport
  wires:
  Sum1/1 -> Scope2/2, Out1/1
  Sum/1 -> Scope4/1, Scope3/2, Mux1/2, Relational Operator1/2, Scope5/1, Relational Operator/1, Mux/3
  3rd harmonic injection/1 -> Sum/2
  Mux/1 -> Scope/1
  Carrier wave +ve/1 -> Scope3/3, Mux1/3, Scope5/2, Relational Operator/2, Mux/1
  Relational Operator/1 -> Sum1/1
  Relational Operator1/1 -> Sum1/2
  Mux1/1 -> Scope2/1
  Carrier wave -ve/1 -> Scope3/1, Mux1/1, Relational Operator1/1, Mux/2
  "Ref Signal "/1 -> Scope1/1, Sum/1

== system transfer_function_calculation/Generator/3 Level Converter2/SPWM Generator/Comparator Phase C ==
  Ref Signal : Inport
  3rd harmonic injection : Sin  Amplitude=Vh  Frequency=314*3  SampleTime=0
  Carrier wave +ve : simulink/Sources/Repeating Sequence  rep_seq_t=.0001*[0 2 4]  rep_seq_y=a*[2 0 2]
  Carrier wave -ve : simulink/Sources/Repeating Sequence  rep_seq_t=.0001*[0 2 4]  rep_seq_y=a*[0 -2 0]
  Mux : Mux  Inputs=3
  Relational Operator : RelationalOperator  Operator=>  OutDataTypeStr=fixdt(1,16)
  Relational Operator1 : RelationalOperator  Operator=>  OutDataTypeStr=boolean
  Scope : Scope
  Scope4 : Scope
  Scope5 : Scope  NumInputPorts=2
  Scope6 : Scope  NumInputPorts=3
  Sum : Sum  Inputs=|++
  Sum1 : Sum  Inputs=|+-
  Out1 : Outport
  wires:
  Sum1/1 -> Out1/1
  Sum/1 -> Scope4/1, Scope6/2, Relational Operator1/2, Scope5/1, Relational Operator/1, Mux/3
  Carrier wave -ve/1 -> Scope6/1, Relational Operator1/1, Mux/2
  Ref Signal/1 -> Sum/1
  3rd harmonic injection/1 -> Sum/2
  Mux/1 -> Scope/1
  Carrier wave +ve/1 -> Scope5/2, Relational Operator/2, Mux/1
  Relational Operator/1 -> Sum1/1
  Relational Operator1/1 -> Sum1/2, Scope6/3

== system transfer_function_calculation/Generator/3 Level Converter2/SPWM Generator/SPWM A ==
  Switching signal : Inport
  Mux : Mux
  S1 : simulink/Logic and Bit Operations/Compare To Zero  relop=>=  OutDataTypeStr=boolean
  S11 : simulink/Logic and Bit Operations/Compare To Zero  relop=<=  OutDataTypeStr=boolean
  "S2 " : simulink/Logic and Bit Operations/Compare To Zero  relop=>  OutDataTypeStr=boolean
  S21 : simulink/Logic and Bit Operations/Compare To Zero  relop=<  OutDataTypeStr=boolean
  Scope : Scope
  Scope1 : Scope  NumInputPorts=2
  Scope2 : Scope  NumInputPorts=2
  Out1 : Outport
  Out2 : Outport  Port=2
  Out3 : Outport  Port=3
  Out4 : Outport  Port=4
  wires:
  S11/1 -> Scope2/1, Mux/3, Out3/1
  S21/1 -> Scope2/2, Mux/4, Out4/1
  Switching signal/1 -> S1/1, S21/1, S11/1, "S2 "/1
  S1/1 -> Scope1/1, Mux/1, Out1/1
  "S2 "/1 -> Scope1/2, Mux/2, Out2/1
  Mux/1 -> Scope/1

== system transfer_function_calculation/Generator/3 Level Converter2/SPWM Generator/SPWM B ==
  In1 : Inport
  Compare To Zero4 : simulink/Logic and Bit Operations/Compare To Zero  relop=>=  OutDataTypeStr=boolean
  Compare To Zero5 : simulink/Logic and Bit Operations/Compare To Zero  relop=>  OutDataTypeStr=boolean
  Compare To Zero6 : simulink/Logic and Bit Operations/Compare To Zero  relop=<=  OutDataTypeStr=boolean
  Compare To Zero7 : simulink/Logic and Bit Operations/Compare To Zero  relop=<  OutDataTypeStr=boolean
  Out1 : Outport
  Out2 : Outport  Port=2
  Out3 : Outport  Port=3
  Out4 : Outport  Port=4
  wires:
  In1/1 -> Compare To Zero5/1, Compare To Zero6/1, Compare To Zero7/1, Compare To Zero4/1
  Compare To Zero4/1 -> Out1/1
  Compare To Zero5/1 -> Out2/1
  Compare To Zero6/1 -> Out3/1
  Compare To Zero7/1 -> Out4/1

== system transfer_function_calculation/Generator/3 Level Converter2/SPWM Generator/SPWM C ==
  In1 : Inport
  Compare To Zero10 : simulink/Logic and Bit Operations/Compare To Zero  relop=<=  OutDataTypeStr=boolean
  Compare To Zero11 : simulink/Logic and Bit Operations/Compare To Zero  relop=<  OutDataTypeStr=boolean
  Compare To Zero8 : simulink/Logic and Bit Operations/Compare To Zero  relop=>=  OutDataTypeStr=boolean
  Compare To Zero9 : simulink/Logic and Bit Operations/Compare To Zero  relop=>  OutDataTypeStr=boolean
  Out1 : Outport
  Out2 : Outport  Port=2
  Out3 : Outport  Port=3
  Out4 : Outport  Port=4
  wires:
  In1/1 -> Compare To Zero10/1, Compare To Zero11/1, Compare To Zero8/1, Compare To Zero9/1
  Compare To Zero10/1 -> Out3/1
  Compare To Zero8/1 -> Out1/1
  Compare To Zero9/1 -> Out2/1
  Compare To Zero11/1 -> Out4/1

== system transfer_function_calculation/Generator/Generator /Parktransformation/Three-phase current ==
  In1 : Inport
  In2 : Inport  Port=2
  Constant3 : Constant  Value=2*pi/3
  Constant4 : Constant  Value=-2*pi/3
  Gain : Gain  Gain=2*pi
  Integrator : Integrator
  Mux : Mux  Inputs=3
  Product : Product
  Sum : Sum  Inputs=|++
  Sum1 : Sum  Inputs=|++
  Trigonometric Function : Trigonometry  Operator=cos
  "abc " : Outport
  wires:
  Constant4/1 -> Sum1/2
  Trigonometric Function/1 -> Product/1
  Gain/1 -> Integrator/1
  In1/1 -> Gain/1
  In2/1 -> Product/2
  Sum/1 -> Mux/2
  Constant3/1 -> Sum/2
  Sum1/1 -> Mux/3
  Mux/1 -> Trigonometric Function/1
  Integrator/1 -> Sum/1, Sum1/1, Mux/1
  Product/1 -> "abc "/1

== system transfer_function_calculation/Generator/Generator /Parktransformation/abc to alpha-beta ==
  abc : Inport
  Demux : Demux  Outputs=3
  Gain : Gain  Gain=1/sqrt(3)
  Mux : Mux  Inputs=2
  Sum : Sum  Inputs=|+-
  "alpha-beta " : Outport
  wires:
  abc/1 -> Demux/1
  Sum/1 -> Gain/1
  Demux/2 -> Sum/1
  Demux/3 -> Sum/2
  Gain/1 -> Mux/2
  Demux/1 -> Mux/1
  Mux/1 -> "alpha-beta "/1

== system transfer_function_calculation/Generator/Generator /Parktransformation/alpha-beta to dq ==
  theta : Inport
  "alpha-beta " : Inport  Port=2
  Demux : Demux  Outputs=2
  Mux : Mux  Inputs=2
  Product{,1..3} (4 alike) : Product
  Sum : Sum  Inputs=|++
  Sum1 : Sum  Inputs=|+-
  Trigonometric Function : Trigonometry  Operator=cos
  Trigonometric Function1 : Trigonometry
  Out1 : Outport
  wires:
  Trigonometric Function1/1 -> Product3/2, Product1/2
  Product/1 -> Sum/1
  Product3/1 -> Sum1/2
  Product2/1 -> Sum1/1
  Sum/1 -> Mux/1
  Demux/1 -> Product3/1, Product/1
  Trigonometric Function/1 -> Product2/2, Product/2
  Demux/2 -> Product2/1, Product1/1
  Sum1/1 -> Mux/2
  Product1/1 -> Sum/2
  Mux/1 -> Out1/1
  "alpha-beta "/1 -> Demux/1
  theta/1 -> Trigonometric Function1/1, Trigonometric Function/1

== system transfer_function_calculation/Generator/Generator Controller /Parktransformation/3phase to ab ==
  In1 : Inport
  Demux : Demux  Outputs=3
  Gain3 : Gain  Gain=1/sqrt(3)
  Mux : Mux  Inputs=2
  Scope : Scope
  Sum1 : Sum  Inputs=|+-
  Out1 : Outport
  wires:
  Mux/1 -> Scope/1, Out1/1
  Demux/2 -> Sum1/1
  Demux/3 -> Sum1/2
  Sum1/1 -> Gain3/1
  In1/1 -> Demux/1
  Demux/1 -> Mux/1
  Gain3/1 -> Mux/2

== system transfer_function_calculation/Generator/Generator Controller /Parktransformation/alpha-beta to dq ==
  theta : Inport
  "alpha-beta " : Inport  Port=2
  Demux : Demux  Outputs=2
  Mux : Mux  Inputs=2
  Product{,1..3} (4 alike) : Product
  Sum : Sum  Inputs=|++
  Sum1 : Sum  Inputs=|+-
  Trigonometric Function : Trigonometry  Operator=cos
  Trigonometric Function1 : Trigonometry
  Out1 : Outport
  wires:
  Trigonometric Function1/1 -> Product3/2, Product1/2
  Product/1 -> Sum/1
  Product3/1 -> Sum1/2
  Product2/1 -> Sum1/1
  Sum/1 -> Mux/1
  Demux/1 -> Product3/1, Product/1
  Trigonometric Function/1 -> Product2/2, Product/2
  Demux/2 -> Product2/1, Product1/1
  Sum1/1 -> Mux/2
  Product1/1 -> Sum/2
  Mux/1 -> Out1/1
  "alpha-beta "/1 -> Demux/1
  theta/1 -> Trigonometric Function1/1, Trigonometric Function/1

== system transfer_function_calculation/Generator/3 Level Converter2/Loss Calculation/Leg A1/Heat Sink (Simscape thermal model) ==
  Ta : Inport
  Conductive Heat Transfer Case 1 to Sink : fl_lib/Thermal/Thermal Elements/Conductive Heat Transfer  area=1 m^2  thickness=1 m  th_cond=1/Rth(1) W/(m*K)  Q_specify=off  Q_priority=High  Q=0 J/s  T_specify=off  T_priority=High  T=0 K
  Convective Heat Transfer Sink-to-Ambient : fl_lib/Thermal/Thermal Elements/Convective Heat Transfer  area=1 m^2  heat_tr_coeff=1/Rth(2) W/(m^2 * K)  Q_specify=off  Q_priority=High  Q=0 J/s  T_specify=off  T_priority=High  T=0 K
  PS2S : Subsystem
  PS2S1 : Subsystem
  S2PS1 : Subsystem
  Scope : Scope
  Scope1 : Scope
  Simscape Solver Configuration : nesl_utility/Solver Configuration  PhysicalDomain=network_engine_domain  SubClassName=solver  LeftPortType=input  RightPortType=generic  Accelerate=off  Tones=[]  Harmonics=[]  SimulateNoise=off  Profile=off  UseLocalSampling=off  EnableSwitchedLinearOptims=on  FrequencyDomain=off  UseCCode=off  RelTol=0.001  AbsTol=1e-06  MinStep=1e-09  ToWorkspace=off  RevertToSquareIcSolve=off  NumHomotopyIterations=100  PhasorMode=off  PhasorModeNumHarmonics=1  OverrideAbsTol=off  DoDC=off  ResidualTolerance=1e-9  UseLocalSolver=on  LocalSolverChoice=NE_TRAPEZOIDAL_ADVANCER  LocalSolverSampleTime=Ts_Control  DoFixedCost=off  MaxNonlinIter=2  MaxModeIter=1  LinearAlgebra=Sparse  DelaysMemoryBudget=1024  AutomaticFiltering=on  FilteringTimeConstant=0.001
  Temperature Sensor : fl_lib/Thermal/Thermal Sensors/Ideal Temperature Sensor
  Temperature Sensor1 : fl_lib/Thermal/Thermal Sensors/Ideal Temperature Sensor
  Temperature Source : fl_lib/Thermal/Thermal Sources/Ideal Temperature Source
  Thermal Reference : fl_lib/Thermal/Thermal Elements/Thermal Reference
  Thermal Reference1 : fl_lib/Thermal/Thermal Elements/Thermal Reference
  Thermal Reference2 : fl_lib/Thermal/Thermal Elements/Thermal Reference
  Thermal Mass (Case 1) : fl_lib/Thermal/Thermal Elements/Thermal Mass  mass=Cth(1) kg  sp_heat=1 J/kg/K  T_specify=on  T_priority=High  T=Tinit degC  Q_specify=off  Q_priority=High  Q=0 J/s
  Thermal Mass (Heatsink) : fl_lib/Thermal/Thermal Elements/Thermal Mass  mass=Cth(2) kg  sp_heat=1 J/kg/K  T_specify=on  T_priority=High  T=Tinit degC  Q_specify=off  Q_priority=High  Q=0 J/s
  H1 : PMIOPort  Port=1  Side=Right
  Tsink : Outport
  wires:
  PS2S/1(Out) -> Tsink/1
  Ta/1 -> Scope/1, S2PS1/1(In)
  PS2S1/1(Out) -> Scope1/1
  connections:
  Temperature Sensor/RConn2 -- PS2S/LConn1
  Temperature Sensor/RConn1 -- Thermal Reference/LConn1
  Simscape Solver Configuration/RConn1 -- Conductive Heat Transfer Case 1 to Sink/RConn1 -- Thermal Mass (Heatsink)/LConn1 -- Convective Heat Transfer Sink-to-Ambient/LConn1 -- Temperature Sensor/LConn1
  Convective Heat Transfer Sink-to-Ambient/RConn1 -- Temperature Sensor1/LConn1 -- Temperature Source/LConn1
  S2PS1/RConn1 -- Temperature Source/RConn1
  Temperature Source/RConn2 -- Thermal Reference1/LConn1
  Conductive Heat Transfer Case 1 to Sink/LConn1 -- Thermal Mass (Case 1)/LConn1 -- H1/RConn1
  Temperature Sensor1/RConn1 -- Thermal Reference2/LConn1
  Temperature Sensor1/RConn2 -- PS2S1/LConn1

== system transfer_function_calculation/Generator/3 Level Converter2/Loss Calculation/Leg A1/Subsystem ==
  In1 : Inport
  In2 : Inport  Port=2
  Bus Creator : Subsystem
  Loss Calculation Unit : Subsystem
  Scope : Scope
  Scope1 : Scope
  Scope2 : Scope
  Conn1 : PMIOPort  Port=1  Side=Left
  Out1 : Outport
  wires:
  Loss Calculation Unit/3(Psw_IGBTs) -> Scope1/1, Bus Creator/3(In3)
  In1/1 -> Loss Calculation Unit/1(From m point of  IGBT1)
  Loss Calculation Unit/1(mQd1) -> Bus Creator/1(In1)
  Loss Calculation Unit/9(Ptot_HB) -> Bus Creator/9(In9)
  Loss Calculation Unit/7(Pcond_diodes) -> Bus Creator/7(In7)
  Loss Calculation Unit/8(Ptot_Diodes) -> Bus Creator/8(In8)
  In2/1 -> Loss Calculation Unit/2(From m point of  IGBT2)
  Loss Calculation Unit/11(TJ_Diodes) -> Bus Creator/11(In11)
  Loss Calculation Unit/10(TJ_IGBT) -> Bus Creator/10(In10)
  Loss Calculation Unit/6(Psw_Diodes) -> Scope2/1, Bus Creator/6(In6)
  Loss Calculation Unit/5(Ptot_IGBTs) -> Bus Creator/5(In5)
  Loss Calculation Unit/2(mQd2) -> Bus Creator/2(In2)
  Bus Creator/1(m) -> Out1/1
  Loss Calculation Unit/4(Pcond_IGBT) -> Bus Creator/4(In4), Scope/1
  Loss Calculation Unit/12(Tcase) -> Bus Creator/12(In12)
  connections:
  Conn1/RConn1 -- Loss Calculation Unit/RConn1

== system transfer_function_calculation/Generator/3 Level Converter2/Loss Calculation/Leg A2/Heat Sink (Simscape thermal model) ==
  Ta : Inport
  Conductive Heat Transfer Case 1 to Sink : fl_lib/Thermal/Thermal Elements/Conductive Heat Transfer  area=1 m^2  thickness=1 m  th_cond=1/Rth(1) W/(m*K)  Q_specify=off  Q_priority=High  Q=0 J/s  T_specify=off  T_priority=High  T=0 K
  Convective Heat Transfer Sink-to-Ambient : fl_lib/Thermal/Thermal Elements/Convective Heat Transfer  area=1 m^2  heat_tr_coeff=1/Rth(2) W/(m^2 * K)  Q_specify=off  Q_priority=High  Q=0 J/s  T_specify=off  T_priority=High  T=0 K
  PS2S : Subsystem
  PS2S1 : Subsystem
  S2PS1 : Subsystem
  Scope : Scope
  Scope1 : Scope
  Simscape Solver Configuration : nesl_utility/Solver Configuration  PhysicalDomain=network_engine_domain  SubClassName=solver  LeftPortType=input  RightPortType=generic  Accelerate=off  Tones=[]  Harmonics=[]  SimulateNoise=off  Profile=off  UseLocalSampling=off  EnableSwitchedLinearOptims=on  FrequencyDomain=off  UseCCode=off  RelTol=0.001  AbsTol=1e-06  MinStep=1e-09  ToWorkspace=off  RevertToSquareIcSolve=off  NumHomotopyIterations=100  PhasorMode=off  PhasorModeNumHarmonics=1  OverrideAbsTol=off  DoDC=off  ResidualTolerance=1e-9  UseLocalSolver=on  LocalSolverChoice=NE_TRAPEZOIDAL_ADVANCER  LocalSolverSampleTime=Ts_Control  DoFixedCost=off  MaxNonlinIter=2  MaxModeIter=1  LinearAlgebra=Sparse  DelaysMemoryBudget=1024  AutomaticFiltering=on  FilteringTimeConstant=0.001
  Temperature Sensor : fl_lib/Thermal/Thermal Sensors/Ideal Temperature Sensor
  Temperature Sensor1 : fl_lib/Thermal/Thermal Sensors/Ideal Temperature Sensor
  Temperature Source : fl_lib/Thermal/Thermal Sources/Ideal Temperature Source
  Thermal Reference : fl_lib/Thermal/Thermal Elements/Thermal Reference
  Thermal Reference1 : fl_lib/Thermal/Thermal Elements/Thermal Reference
  Thermal Reference2 : fl_lib/Thermal/Thermal Elements/Thermal Reference
  Thermal Mass (Case 1) : fl_lib/Thermal/Thermal Elements/Thermal Mass  mass=Cth(1) kg  sp_heat=1 J/kg/K  T_specify=on  T_priority=High  T=Tinit degC  Q_specify=off  Q_priority=High  Q=0 J/s
  Thermal Mass (Heatsink) : fl_lib/Thermal/Thermal Elements/Thermal Mass  mass=Cth(2) kg  sp_heat=1 J/kg/K  T_specify=on  T_priority=High  T=Tinit degC  Q_specify=off  Q_priority=High  Q=0 J/s
  H1 : PMIOPort  Port=1  Side=Right
  Tsink : Outport
  wires:
  PS2S1/1(Out) -> Scope1/1
  Ta/1 -> S2PS1/1(In), Scope/1
  PS2S/1(Out) -> Tsink/1
  connections:
  Temperature Sensor1/RConn2 -- PS2S1/LConn1
  Temperature Sensor1/RConn1 -- Thermal Reference2/LConn1
  H1/RConn1 -- Thermal Mass (Case 1)/LConn1 -- Conductive Heat Transfer Case 1 to Sink/LConn1
  Temperature Source/RConn2 -- Thermal Reference1/LConn1
  S2PS1/RConn1 -- Temperature Source/RConn1
  Temperature Source/LConn1 -- Temperature Sensor1/LConn1 -- Convective Heat Transfer Sink-to-Ambient/RConn1
  Temperature Sensor/LConn1 -- Convective Heat Transfer Sink-to-Ambient/LConn1 -- Thermal Mass (Heatsink)/LConn1 -- Conductive Heat Transfer Case 1 to Sink/RConn1 -- Simscape Solver Configuration/RConn1
  Temperature Sensor/RConn1 -- Thermal Reference/LConn1
  Temperature Sensor/RConn2 -- PS2S/LConn1

== system transfer_function_calculation/Generator/3 Level Converter2/Loss Calculation/Leg A2/Subsystem ==
  In1 : Inport
  In2 : Inport  Port=2
  Bus Creator : Subsystem
  Loss Calculation Unit : Subsystem
  Scope : Scope
  Scope1 : Scope
  Scope2 : Scope
  Conn1 : PMIOPort  Port=1  Side=Left
  Out1 : Outport
  wires:
  Loss Calculation Unit/12(Tcase) -> Bus Creator/12(In12)
  Loss Calculation Unit/4(Pcond_IGBT) -> Scope/1, Bus Creator/4(In4)
  Bus Creator/1(m) -> Out1/1
  Loss Calculation Unit/2(mQd2) -> Bus Creator/2(In2)
  Loss Calculation Unit/5(Ptot_IGBTs) -> Bus Creator/5(In5)
  Loss Calculation Unit/6(Psw_Diodes) -> Bus Creator/6(In6), Scope2/1
  Loss Calculation Unit/10(TJ_IGBT) -> Bus Creator/10(In10)
  Loss Calculation Unit/11(TJ_Diodes) -> Bus Creator/11(In11)
  In2/1 -> Loss Calculation Unit/2(QD2)
  Loss Calculation Unit/8(Ptot_Diodes) -> Bus Creator/8(In8)
  Loss Calculation Unit/7(Pcond_diodes) -> Bus Creator/7(In7)
  Loss Calculation Unit/9(Ptot_HB) -> Bus Creator/9(In9)
  Loss Calculation Unit/1(mQd1) -> Bus Creator/1(In1)
  In1/1 -> Loss Calculation Unit/1(QD1)
  Loss Calculation Unit/3(Psw_IGBTs) -> Bus Creator/3(In3), Scope1/1
  connections:
  Conn1/RConn1 -- Loss Calculation Unit/RConn1

== system transfer_function_calculation/Generator/3 Level Converter2/Loss Calculation/Leg B1/Heat Sink (Simscape thermal model) ==
  Ta : Inport
  Conductive Heat Transfer Case 1 to Sink : fl_lib/Thermal/Thermal Elements/Conductive Heat Transfer  area=1 m^2  thickness=1 m  th_cond=1/Rth(1) W/(m*K)  Q_specify=off  Q_priority=High  Q=0 J/s  T_specify=off  T_priority=High  T=0 K
  Convective Heat Transfer Sink-to-Ambient : fl_lib/Thermal/Thermal Elements/Convective Heat Transfer  area=1 m^2  heat_tr_coeff=1/Rth(2) W/(m^2 * K)  Q_specify=off  Q_priority=High  Q=0 J/s  T_specify=off  T_priority=High  T=0 K
  PS2S : Subsystem
  PS2S1 : Subsystem
  S2PS1 : Subsystem
  Scope : Scope
  Scope1 : Scope
  Simscape Solver Configuration : nesl_utility/Solver Configuration  PhysicalDomain=network_engine_domain  SubClassName=solver  LeftPortType=input  RightPortType=generic  Accelerate=off  Tones=[]  Harmonics=[]  SimulateNoise=off  Profile=off  UseLocalSampling=off  EnableSwitchedLinearOptims=on  FrequencyDomain=off  UseCCode=off  RelTol=0.001  AbsTol=1e-06  MinStep=1e-09  ToWorkspace=off  RevertToSquareIcSolve=off  NumHomotopyIterations=100  PhasorMode=off  PhasorModeNumHarmonics=1  OverrideAbsTol=off  DoDC=off  ResidualTolerance=1e-9  UseLocalSolver=on  LocalSolverChoice=NE_TRAPEZOIDAL_ADVANCER  LocalSolverSampleTime=Ts_Control  DoFixedCost=off  MaxNonlinIter=2  MaxModeIter=1  LinearAlgebra=Sparse  DelaysMemoryBudget=1024  AutomaticFiltering=on  FilteringTimeConstant=0.001
  Temperature Sensor : fl_lib/Thermal/Thermal Sensors/Ideal Temperature Sensor
  Temperature Sensor1 : fl_lib/Thermal/Thermal Sensors/Ideal Temperature Sensor
  Temperature Source : fl_lib/Thermal/Thermal Sources/Ideal Temperature Source
  Thermal Reference : fl_lib/Thermal/Thermal Elements/Thermal Reference
  Thermal Reference1 : fl_lib/Thermal/Thermal Elements/Thermal Reference
  Thermal Reference2 : fl_lib/Thermal/Thermal Elements/Thermal Reference
  Thermal Mass (Case 1) : fl_lib/Thermal/Thermal Elements/Thermal Mass  mass=Cth(1) kg  sp_heat=1 J/kg/K  T_specify=on  T_priority=High  T=Tinit degC  Q_specify=off  Q_priority=High  Q=0 J/s
  Thermal Mass (Heatsink) : fl_lib/Thermal/Thermal Elements/Thermal Mass  mass=Cth(2) kg  sp_heat=1 J/kg/K  T_specify=on  T_priority=High  T=Tinit degC  Q_specify=off  Q_priority=High  Q=0 J/s
  H1 : PMIOPort  Port=1  Side=Right
  Tsink : Outport
  wires:
  PS2S/1(Out) -> Tsink/1
  Ta/1 -> Scope/1, S2PS1/1(In)
  PS2S1/1(Out) -> Scope1/1
  connections:
  Temperature Sensor/RConn2 -- PS2S/LConn1
  Temperature Sensor/RConn1 -- Thermal Reference/LConn1
  Simscape Solver Configuration/RConn1 -- Conductive Heat Transfer Case 1 to Sink/RConn1 -- Thermal Mass (Heatsink)/LConn1 -- Convective Heat Transfer Sink-to-Ambient/LConn1 -- Temperature Sensor/LConn1
  Convective Heat Transfer Sink-to-Ambient/RConn1 -- Temperature Sensor1/LConn1 -- Temperature Source/LConn1
  S2PS1/RConn1 -- Temperature Source/RConn1
  Temperature Source/RConn2 -- Thermal Reference1/LConn1
  Conductive Heat Transfer Case 1 to Sink/LConn1 -- Thermal Mass (Case 1)/LConn1 -- H1/RConn1
  Temperature Sensor1/RConn1 -- Thermal Reference2/LConn1
  Temperature Sensor1/RConn2 -- PS2S1/LConn1
